simulink model "model_TS_Lab_8a"  (Simulink 7.2)
settings: Solver=ode4  StartTime=0.0  StopTime=czas  FixedStep=0.001  RelTol=1e-3
values from neighbouring files (symbols this model uses):
  a = -2    [lab8.m]    (also in skrypt_TS_Lab_8a.m = -1)
  A_u = 5    [skrypt_TS_Lab_8a.m]
  A_ud = 1.5    [skrypt_TS_Lab_8a.m]
  b = 2    [lab8.m]    (also in skrypt_TS_Lab_8a.m = 1)
  c = 1    [lab8.m]    (also in skrypt_TS_Lab_8a.m)
  f_u = 0.05    [skrypt_TS_Lab_8a.m]
  f_ud = 100    [skrypt_TS_Lab_8a.m]
  Licznik = Ko.num{1}    [skrypt_TS_Lab_8a.m]
  Mianownik = Ko.den{1}    [skrypt_TS_Lab_8a.m]
settings Model: Creator=WiErZgI  LastModifiedBy=Lucas
settings DataIOCC: LimitDataPoints=off

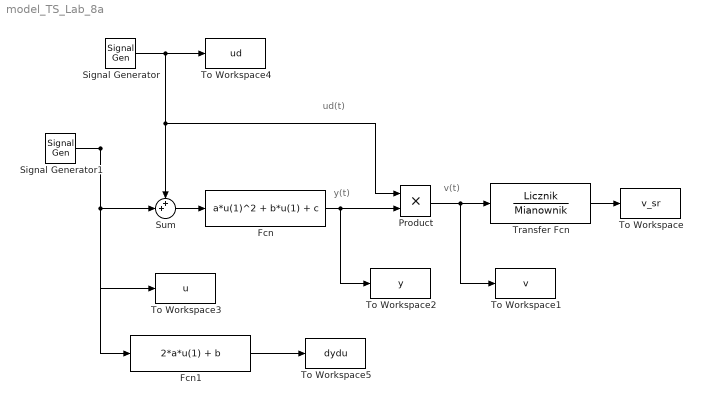
== system model_TS_Lab_8a ==
  note: v(t)
  note: y(t)
  note: ud(t)
  Fcn : Fcn  Expr=a*u(1)^2 + b*u(1) + c
  Fcn1 : Fcn  Expr=2*a*u(1) + b
  Product : Product  RndMeth=Zero
  Signal Generator : SignalGenerator  Amplitude=A_ud  Frequency=f_ud
  Signal Generator1 : SignalGenerator  WaveForm=square  Amplitude=A_u  Frequency=f_u
  Sum : Sum  Inputs=++|
  To Workspace : ToWorkspace  VariableName=v_sr  SampleTime=-1  SaveFormat=Array
  To Workspace1 : ToWorkspace  VariableName=v  SampleTime=-1  SaveFormat=Array
  To Workspace2 : ToWorkspace  VariableName=y  SampleTime=-1  SaveFormat=Array
  To Workspace3 : ToWorkspace  VariableName=u  SampleTime=-1  SaveFormat=Array
  To Workspace4 : ToWorkspace  VariableName=ud  SampleTime=-1  SaveFormat=Array
  To Workspace5 : ToWorkspace  VariableName=dydu  SampleTime=-1  SaveFormat=Array
  Transfer Fcn : TransferFcn  Numerator=Licznik  Denominator=Mianownik
  wires:
  Signal Generator/1 -> Sum/1, Product/1, To Workspace4/1
  Sum/1 -> Fcn/1
  Fcn/1 -> Product/2, To Workspace2/1
  Product/1 -> Transfer Fcn/1, To Workspace1/1
  Transfer Fcn/1 -> To Workspace/1
  Fcn1/1 -> To Workspace5/1
  Signal Generator1/1 -> To Workspace3/1, Sum/2, Fcn1/1
